simulink model "first_model"  (R2015b)
settings: Solver=FixedStepAuto  StartTime=0.0  StopTime=30  FixedStep=1  RelTol=1e-3
model workspace (MAT data in the model file):
  SYS_DEL = Simulink.Parameter
  SYS_DEL.Value = 8
  SYS_DEL.DataType = 'auto'
  SYS_DEL.Units = 'auto'
libraries: simulink x2
settings Model: Creator=koprek_w  LastModifiedBy=koprek_w

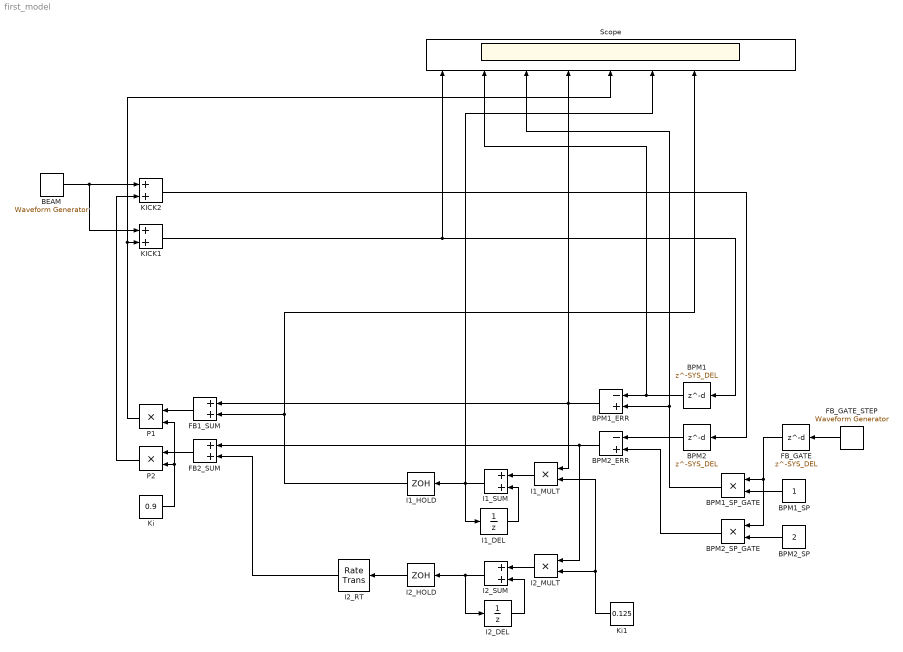
== system first_model ==
  BEAM : simulink/Sources/Waveform Generator  OutMin=[]  OutMax=[]  OutDataTypeStr=double  SelectedSignal=1  Signals=step(0,0,0.8)  BlockNames=MultiportSwitch_57682597a0114c1  SampleTime=1
  BPM1 : Delay  DelayLength=SYS_DEL
  BPM1_ERR : Sum  Inputs=-+
  BPM1_SP : Constant
  BPM1_SP_GATE : Product
  BPM2 : Delay  DelayLength=SYS_DEL
  BPM2_ERR : Sum  Inputs=-+
  BPM2_SP : Constant  Value=2
  BPM2_SP_GATE : Product
  FB1_SUM : Sum
  FB2_SUM : Sum
  FB_GATE : Delay  DelayLength=SYS_DEL
  FB_GATE_STEP : simulink/Sources/Waveform Generator  OutMin=[]  OutMax=[]  OutDataTypeStr=double  SelectedSignal=1  Signals=step(0,0,1)  BlockNames=MultiportSwitch_a39c8a027058463  SampleTime=1
  I1_DEL : UnitDelay  SampleTime=-1
  I1_HOLD : ZeroOrderHold  SampleTime=-1
  I1_MULT : Product
  I1_SUM : Sum
  I2_DEL : UnitDelay  SampleTime=-1
  I2_HOLD : ZeroOrderHold  SampleTime=SYS_DEL
  I2_MULT : Product
  I2_RT : RateTransition  OutPortSampleTimeOpt=Inherit
  I2_SUM : Sum
  KICK1 : Sum
  KICK2 : Sum
  Ki : Constant  Value=0.9
  Ki1 : Constant  Value=0.125
  P1 : Product
  P2 : Product
  Scope : Scope  NumInputPorts=9
  wires:
  BEAM/1 -> KICK1/1, KICK2/1
  KICK1/1 -> BPM1/1, Scope/1
  KICK2/1 -> BPM2/1
  Ki/1 -> P1/2, P2/2
  P1/1 -> Scope/5, KICK1/2
  P2/1 -> KICK2/2
  BPM1/1 -> BPM1_ERR/1, Scope/2
  BPM2/1 -> BPM2_ERR/1
  BPM1_ERR/1 -> Scope/4, FB1_SUM/1, I1_MULT/1
  BPM2_ERR/1 -> I2_MULT/1, FB2_SUM/1
  FB_GATE_STEP/1 -> FB_GATE/1
  FB_GATE/1 -> BPM2_SP_GATE/1, BPM1_SP_GATE/1
  BPM1_SP_GATE/1 -> BPM1_ERR/2, Scope/3
  BPM2_SP_GATE/1 -> BPM2_ERR/2
  BPM2_SP/1 -> BPM2_SP_GATE/2
  BPM1_SP/1 -> BPM1_SP_GATE/2
  I1_SUM/1 -> Scope/6, I1_HOLD/1, I1_DEL/1
  I1_MULT/1 -> I1_SUM/1
  I2_MULT/1 -> I2_SUM/1
  Ki1/1 -> I2_MULT/2, I1_MULT/2
  I1_DEL/1 -> I1_SUM/2
  I2_SUM/1 -> I2_DEL/1, I2_HOLD/1
  I2_DEL/1 -> I2_SUM/2
  FB1_SUM/1 -> P1/1
  FB2_SUM/1 -> P2/1
  I1_HOLD/1 -> Scope/7, FB1_SUM/2
  I2_HOLD/1 -> I2_RT/1
  I2_RT/1 -> FB2_SUM/2
